simulink model "Drone_Model"  (R2019b)
settings: Solver=VariableStepAuto  StartTime=0.0  StopTime=1  RelTol=1e-3
values from neighbouring files (symbols this model uses):
  A = double(round(subs(J_x,   [states, inputs], [trim_state, trim_input])*1000)/1000)    [state_decoupling.m]
  A_double = [0 1; 0 0]    [kalman_matrices_calculator.m]
  A_s_double = eval(subs(Ad_double,Ts))    [kalman_matrices_calculator.m]
  A_s_single = eval(subs(Ad_single,Ts))    [kalman_matrices_calculator.m]
  A_single = [0]    [kalman_matrices_calculator.m]
  Aaileron = A(5:8,5:8)    [state_decoupling.m]
  Aelevator = A(1:4,1:4)    [state_decoupling.m]
  Arudder = A(11:12,11:12)    [state_decoupling.m]
  Athrust = A(9:10,9:10)    [state_decoupling.m]
  B = B*MotorMix    [state_decoupling.m]
  B_double = [0; 1]    [kalman_matrices_calculator.m]
  B_s_double = eval(subs(Bd_double,Ts))    [kalman_matrices_calculator.m]
  B_s_single = eval(subs(Bd_single,Ts))    [kalman_matrices_calculator.m]
  B_single = [1]    [kalman_matrices_calculator.m]
  Baileron = B(5:8,3)    [state_decoupling.m]
  Belevator = B(1:4,2)    [state_decoupling.m]
  Brudder = B(11:12,4)    [state_decoupling.m]
  Bthrust = B(9:10,1)    [state_decoupling.m]
  C = double(round(subs(J_y,   [states, inputs], [trim_state, trim_input])*1000)/1000)    [state_decoupling.m]
  C_double = [1 0]    [kalman_matrices_calculator.m]
  C_P = 0.041    [state_decoupling.m]
  C_rollpitch = rho*prop_dia^4*prop_dist/sqrt(2)*[                 1  -1  -1   1 ;                 1   1  -1  -1 ;                 0   0   0   0 ; ]    [state_decoupling.m]
  C_single = [1]    [kalman_matrices_calculator.m]
  C_T = [0.069075;4.95e-05]    [state_decoupling.m]
  C_yaw = rho*prop_dia^5/(2*pi)*[                 0   0   0   0 ;                 0   0   0   0 ;                -1   1  -1   1 ; ]    [state_decoupling.m]
  Caileron = [0 1 0 0; 0 0 0 1]    [state_decoupling.m]
  Celevator = [0 1 0 0; 0 0 0 1]    [state_decoupling.m]
  Crudder = [0 1]    [state_decoupling.m]
  Cthrust = [ 1 0; 0 0]    [state_decoupling.m]
  D = D*MotorMix    [state_decoupling.m]
  D_double = [0]    [kalman_matrices_calculator.m]
  D_single = [0]    [kalman_matrices_calculator.m]
  Daileron = [0 ; 0]    [state_decoupling.m]
  Delevator = [0 ; 0]    [state_decoupling.m]
  Drudder = 0    [state_decoupling.m]
  Dthrust = [0 ; D(4,1)]    [state_decoupling.m]
  g = [0;0;UAV_mass*9.81]    [state_decoupling.m]
  J = [      Jxx   0   0 ;       0   Jyy  0 ;       0    0  Jzz; ]    [state_decoupling.m]
  Jinv = inv(J)    [state_decoupling.m]
  L_double = lqe(A_double, G_double, C_double, q_double, r_double, 0)    [kalman_matrices_calculator.m]
  L_single = lqe(A_single, G_single, C_single, q_single, r_single, 0)    [kalman_matrices_calculator.m]
  measurement_noise = 0.1    [kalman_matrices_calculator.m]
  MotorMix = [                 1  1  1 -1 ;                 1  1 -1  1 ;                 1 -1 -1 -1 ;                 1 -1  1  1 ; ]    [state_decoupling.m]
  omega_c = 2*pi*20    (= 125.663706144)    [kalman_matrices_calculator.m]
  process_noise = 0.05    [kalman_matrices_calculator.m]
  Prop_H = 2*pi*Jprop*[               0  0  0  0 ;               0  0  0  0 ;               1 -1  1 -1 ; ]    [state_decoupling.m]
  q_single = cov(out.In_Out_Data{1}.Values.Data)*10000000000000    [kalman_matrices_calculator.m]
  r_single = cov(out.In_Out_Data{2}.Values.Data)    [kalman_matrices_calculator.m]
  Thrust_Sum = rho*prop_dia^4*[                 0   0   0   0 ;                 0   0   0   0 ;                -1  -1  -1  -1 ; ]    [state_decoupling.m]
  trim_input = [293,293,293,293]    [state_decoupling.m]
  trim_state = [0,0,0,0,0,0,0,0,0,0,0,0]    [state_decoupling.m]
  Ts = 0.005    [kalman_matrices_calculator.m]
  UAV_mass = 0.068    [state_decoupling.m]
undefined symbols (not defined in the file or in its folder): DiscIntNeverNeededParam, Discrete, Time
libraries: ctrlSharedLib x10, simulink x3, vrlib x3, dspmtrx3 x1
settings Model: Creator=crbon  LastModifiedBy=Chris

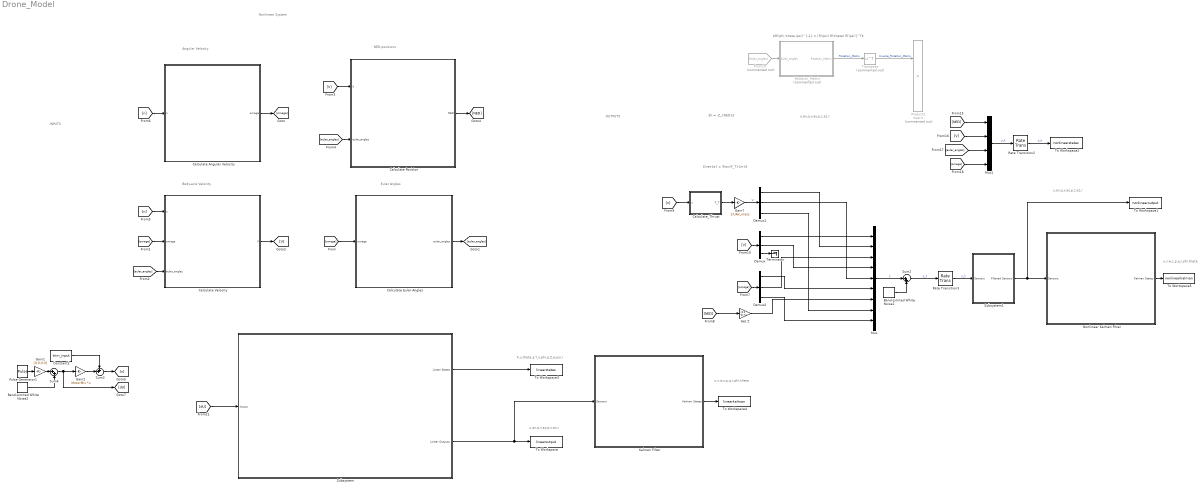
== system Drone_Model ==
  note: X,u,theta,q,Y,v,phi,p,Z,w,psi,r
  note: Nonlinear System
  note: Euler Angles
  note: NED positions
  note: $\vec{a} = \frac{F_T}{m}$
  note: $h = -Z_{NED}$
  note: OUTPUTS
  note: INPUTS
  note: Angular Velocity
  note: Body-axis Velocity
  note: u,ax,q,v,ay,p,z,az,r
  note: u,v,w,z,p,q,r,phi,theta
  note: u,ax,q,v,ay,p,z,az,r
  note: $R(\phi,\theta,\psi)^{-1} = [R(\psi) R(\theta) R(\psi)]^T$
  note: u,v,w,z,p,q,r,phi,theta
  note: u,ax,q,v,ay,p,z,az,r
  Band-Limited White Noise1 : simulink/Sources/Band-Limited White Noise  Cov=measurement_noise*ones(9,1)  Ts=0.05  seed=[11;12;13;14;15;16;17;18;19]
  Band-Limited White Noise2 : simulink/Sources/Band-Limited White Noise  Cov=process_noise*ones(4,1)  Ts=0.05  seed=[1;2;3;4]
  Calculate Angular Velocity : Subsystem
  Calculate Euler Angles : Subsystem
  Calculate Position : Subsystem
  Calculate Velocity : Subsystem
  Calculate_Thrust : Subsystem
  Constant2 : Constant  Value=trim_input
  Demux : Demux  Outputs=3
  Demux1 : Demux  Outputs=3
  Demux2 : Demux  Outputs=3
  From19 : From  Commented=on  GotoTag=euler_angles
  Gain1 : Gain  Gain=[0;0;0;0]
      settings: AttributesFormatString=%<Gain>
  Gain2 : Gain  Gain=MotorMix  Multiplication=Matrix(K*u)
      settings: AttributesFormatString=%<Gain>
  Gain7 : Gain  Gain=1/UAV_mass
      settings: AttributesFormatString=%<Gain>
  Get Z : Gain  Gain=[0 0 -1]  Multiplication=Matrix(K*u)
  Kalman Filter : Subsystem
  Mux : Mux  Inputs=9
  Mux1 : Mux
  Nonlinear Kalman Filter : Subsystem
  Product2 : Product  Commented=on  Multiplication=Matrix(*)
  Pulse Generator1 : DiscretePulseGenerator  PulseType=Time based  Amplitude=0.05  Period=10  PulseWidth=40  PhaseDelay=1
  Rate Transition2 : RateTransition  OutPortSampleTime=0.005
  Rate Transition3 : RateTransition  OutPortSampleTime=0.005
  Rotation_Matrix : Subsystem  Commented=on
  Subsystem : Subsystem
  Subsystem1 : Subsystem
  Sum2 : Sum  Inputs=|++
  Sum3 : Sum  Inputs=++|
  Sum4 : Sum  Inputs=|++
  Terminator : Terminator
  To Workspace : ToWorkspace  VariableName=linearoutput  SaveFormat=Timeseries  SampleTime=-1
  To Workspace1 : ToWorkspace  VariableName=nonlinearoutput  SaveFormat=Timeseries  SampleTime=-1
  To Workspace2 : ToWorkspace  VariableName=nonlinearstates  SaveFormat=Timeseries  SampleTime=-1
  To Workspace3 : ToWorkspace  VariableName=linearstates  SaveFormat=Timeseries  SampleTime=-1
  To Workspace4 : ToWorkspace  VariableName=linearkalman  SaveFormat=Timeseries  SampleTime=-1
  To Workspace5 : ToWorkspace  VariableName=nonlinearkalman  SaveFormat=Timeseries  SampleTime=-1
  Transpose : Math  Commented=on  Operator=transpose  SignedPower=off  SaturateOnIntegerOverflow=on
  wires:
  [omega] -> Calculate Euler Angles/1(omega)
  Calculate Angular Velocity/1(omega) -> [omega]
  [omega] -> Calculate Velocity/2(omega)
  Calculate Euler Angles/1(euler_angles) -> [euler_angles]
  [euler_angles] -> Calculate Velocity/3(euler_angles)
  Calculate Velocity/1(V) -> [V]
  [V] -> Calculate Position/1("V ")
  [euler_angles] -> Calculate Position/2(euler_angles)
  [n] -> Calculate Velocity/1(n)
  [n] -> Calculate Angular Velocity/1(n)
  Calculate Position/1(NED) -> [NED]
  [NED] -> Get Z/1
  Get Z/1 -> Mux/7
  [dU] -> Subsystem/1("Inputs ")
  Subsystem/1(Linear States) -> To Workspace3/1
  Subsystem/2(Linear Outputs) -> Kalman Filter/1(Sensors), To Workspace/1
  Kalman Filter/1(Kalman States) -> To Workspace4/1
  Rotation_Matrix/1(Rotation_Matrix) -> Transpose/1  "Rotation_Matrix"
  From19/1 -> Rotation_Matrix/1("euler_angles ")
  Transpose/1 -> Product2/1  "Inverse_Rotation_Matrix"
  Calculate_Thrust/1(F_T) -> Gain7/1
  [n] -> Calculate_Thrust/1(n)
  Gain7/1 -> Demux1/1  "V"
  [NED] -> Mux1/1
  [euler_angles] -> Mux1/3
  [omega] -> Mux1/4
  [V] -> Mux1/2
  [V] -> Demux/1
  Demux/3 -> Terminator/1
  Demux/1 -> Mux/1
  Demux/2 -> Mux/4
  Demux1/1 -> Mux/2
  Demux1/2 -> Mux/5
  Demux1/3 -> Mux/8
  [omega] -> Demux2/1
  Demux2/1 -> Mux/6
  Demux2/2 -> Mux/3
  Demux2/3 -> Mux/9
  Nonlinear Kalman Filter/1(Kalman States) -> To Workspace5/1
  Mux1/1 -> Rate Transition2/1  "y_k"
  Sum2/1 -> Rate Transition3/1  "y_k"
  Mux/1 -> Sum2/1  "y"
  Rate Transition2/1 -> To Workspace2/1  "y_k"
  Rate Transition3/1 -> Subsystem1/1(Sensors)  "y_k"
  Band-Limited White Noise1/1 -> Sum2/2
  Subsystem1/1(Filtered Sensors) -> Nonlinear Kalman Filter/1(Sensors), To Workspace1/1
  Gain1/1 -> Sum4/1
  Band-Limited White Noise2/1 -> Sum4/2
  Pulse Generator1/1 -> Gain1/1
  Gain2/1 -> Sum3/2
  Sum3/1 -> [n]
  Sum4/1 -> Gain2/1, [dU]
  Constant2/1 -> Sum3/1

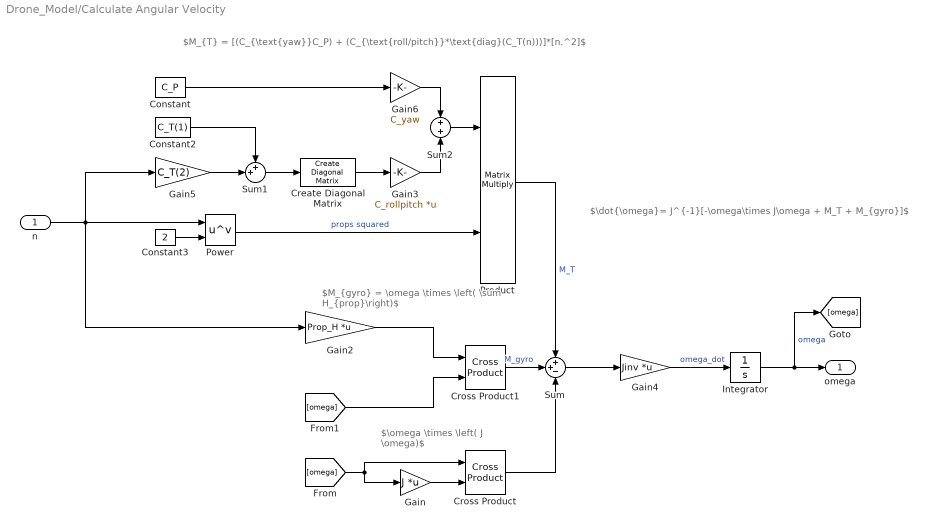
== system Drone_Model/Calculate Angular Velocity ==
  note: $M_{gyro} = \omega \times \left( \sum H_{prop}\right)$
  note: $\dot{\omega}= J^{-1}[-\omega\times J\omega + M_T + M_{gyro}]$
  note: $\omega \times \left( J \omega)$
  note: $M_{T} = [(C_{\text{yaw}}C_P) + (C_{\text{roll/pitch}}*\text{diag}(C_T(n)))]*[n.^2]$
  n : Inport
  Constant : Constant  Value=C_P
  Constant2 : Constant  Value=C_T(1)
  Constant3 : Constant  Value=2
  Create Diagonal Matrix : dspmtrx3/Create Diagonal Matrix
      settings: SourceProductName=DSP System Toolbox  SourceProductBaseCode=DS
  Cross Product : vrlib/Utilities/Cross Product
      settings: SourceProductName=Simulink
  Cross Product1 : vrlib/Utilities/Cross Product
      settings: SourceProductName=Simulink
  Gain : Gain  Gain=J  Multiplication=Matrix(K*u)
  Gain2 : Gain  Gain=Prop_H  Multiplication=Matrix(K*u)
  Gain3 : Gain  Gain=C_rollpitch  Multiplication=Matrix(K*u)
      settings: AttributesFormatString=%<Gain>
  Gain4 : Gain  Gain=Jinv  Multiplication=Matrix(K*u)
      settings: AttributesFormatString=%<Gain>
  Gain5 : Gain  Gain=C_T(2)
  Gain6 : Gain  Gain=C_yaw
      settings: AttributesFormatString=%<Gain>
  Integrator : Integrator  InitialCondition=[0;0;0]
  Power : Math  Operator=pow  SignedPower=off  SaturateOnIntegerOverflow=on
  Product : Product  Multiplication=Matrix(*)
  Sum : Sum  Inputs=++-
  Sum1 : Sum  Inputs=++|
  Sum2 : Sum  Inputs=+|+
  omega : Outport
  wires:
  Sum/1 -> Gain4/1
  [omega] -> Gain/1, Cross Product/1
  Cross Product/1 -> Sum/3
  [omega] -> Cross Product1/2
  Gain2/1 -> Cross Product1/1
  Cross Product1/1 -> Sum/2  "M_gyro"
  Gain4/1 -> Integrator/1  "omega_dot"
  Gain/1 -> Cross Product/2
  Integrator/1 -> [omega], omega/1  "omega"
  Product/1 -> Sum/1  "M_T"
  Create Diagonal Matrix/1 -> Gain3/1
  Sum2/1 -> Product/1
  Sum1/1 -> Create Diagonal Matrix/1
  Constant/1 -> Gain6/1
  Power/1 -> Product/2  "props squared"
  Gain6/1 -> Sum2/1
  Gain5/1 -> Sum1/2
  Gain3/1 -> Sum2/2
  n/1 -> Gain2/1, Power/1, Gain5/1
  Constant2/1 -> Sum1/1
  Constant3/1 -> Power/2

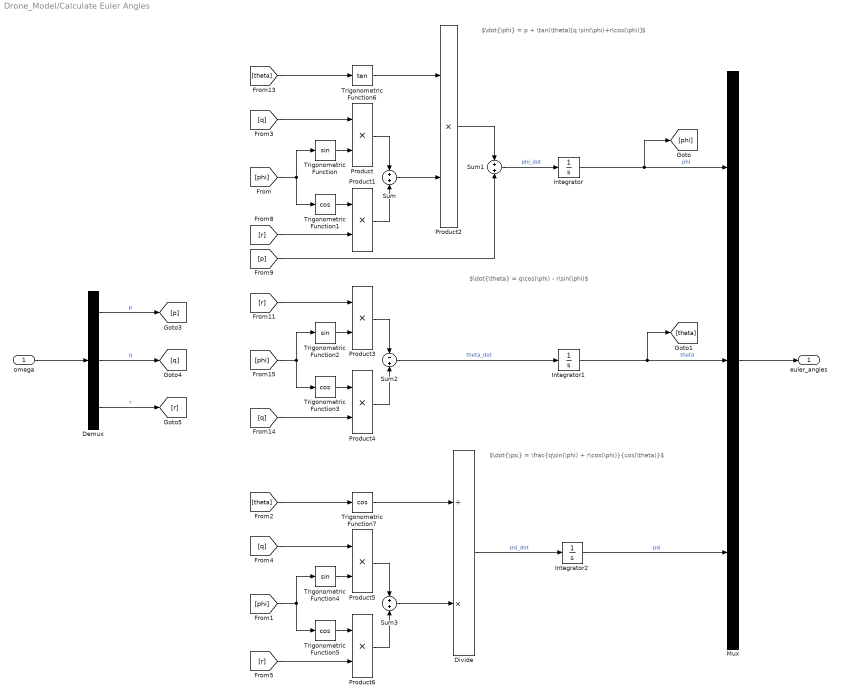
== system Drone_Model/Calculate Euler Angles ==
  note: $\dot{\phi} = p + \tan(\theta)[q \sin(\phi)+r\cos(\phi)]$
  note: $\dot{\theta} = q\cos(\phi) - r\sin(\phi)$
  note: $\dot{\psi} = \frac{q\sin(\phi) + r\cos(\phi)}{cos(\theta)}$
  omega : Inport
  Demux : Demux  Outputs=3
  Divide : Product  Inputs=/*
  Integrator : Integrator
  Integrator1 : Integrator
  Integrator2 : Integrator
  Mux : Mux  Inputs=3
  Product{,1..6} (7 alike) : Product
  Sum : Sum  Inputs=+|+
  Sum1 : Sum  Inputs=+|+
  Sum2 : Sum  Inputs=-|+
  Sum3 : Sum  Inputs=+|+
  Trigonometric Function : Trigonometry
  Trigonometric Function{1,3,5,7} (4 alike) : Trigonometry  Operator=cos
  Trigonometric Function2 : Trigonometry
  Trigonometric Function4 : Trigonometry
  Trigonometric Function6 : Trigonometry  Operator=tan
  euler_angles : Outport
  wires:
  Trigonometric Function7/1 -> Divide/1
  Product1/1 -> Sum/2
  Product6/1 -> Sum3/2
  Trigonometric Function/1 -> Product/2
  Product5/1 -> Sum3/1
  [theta] -> Trigonometric Function7/1
  Trigonometric Function6/1 -> Product2/1
  [r] -> Product6/2
  [theta] -> Trigonometric Function6/1
  Integrator1/1 -> [theta], Mux/2  "theta"
  Trigonometric Function4/1 -> Product5/2
  [q] -> Product4/2
  Demux/3 -> [r]  "r"
  Divide/1 -> Integrator2/1  "psi_dot"
  Integrator2/1 -> Mux/3  "psi"
  [q] -> Product5/1
  Product4/1 -> Sum2/2
  [q] -> Product/1
  [phi] -> Trigonometric Function4/1, Trigonometric Function5/1
  Sum2/1 -> Integrator1/1  "theta_dot"
  Trigonometric Function5/1 -> Product6/1
  Trigonometric Function3/1 -> Product4/1
  [r] -> Product3/1
  Integrator/1 -> [phi], Mux/1  "phi"
  Sum3/1 -> Divide/2
  Product3/1 -> Sum2/1
  [phi] -> Trigonometric Function2/1, Trigonometric Function3/1
  Demux/1 -> [p]  "p"
  Product2/1 -> Sum1/1
  [r] -> Product1/2
  Trigonometric Function1/1 -> Product1/1
  [phi] -> Trigonometric Function1/1, Trigonometric Function/1
  omega/1 -> Demux/1
  Product/1 -> Sum/1
  Demux/2 -> [q]  "q"
  Sum/1 -> Product2/2
  Mux/1 -> euler_angles/1
  Sum1/1 -> Integrator/1  "phi_dot"
  [p] -> Sum1/2
  Trigonometric Function2/1 -> Product3/2

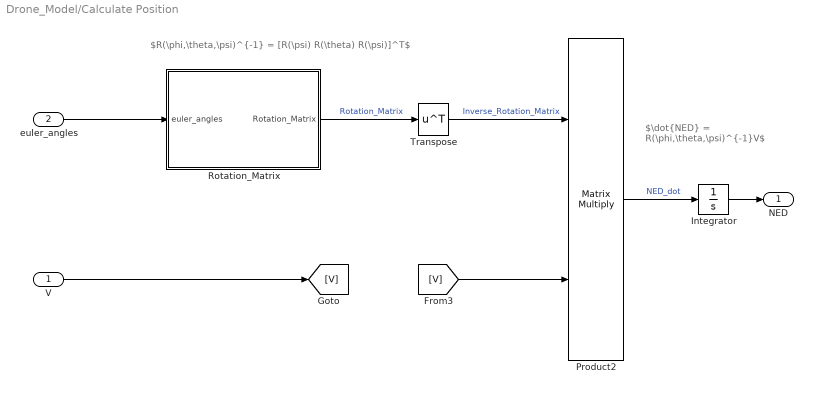
== system Drone_Model/Calculate Position ==
  note: $R(\phi,\theta,\psi)^{-1} = [R(\psi) R(\theta) R(\psi)]^T$
  note: $\dot{NED} = R(\phi,\theta,\psi)^{-1}V$
  "V " : Inport
  euler_angles : Inport  Port=2
  Integrator : Integrator  InitialCondition=[0;0;0]
  Product2 : Product  Multiplication=Matrix(*)
  Rotation_Matrix : Subsystem
  Transpose : Math  Operator=transpose  SignedPower=off  SaturateOnIntegerOverflow=on
  NED : Outport
  wires:
  Product2/1 -> Integrator/1  "NED_dot"
  "V "/1 -> [V]
  Rotation_Matrix/1(Rotation_Matrix) -> Transpose/1  "Rotation_Matrix"
  Transpose/1 -> Product2/1  "Inverse_Rotation_Matrix"
  [V] -> Product2/2
  euler_angles/1 -> Rotation_Matrix/1("euler_angles ")
  Integrator/1 -> NED/1

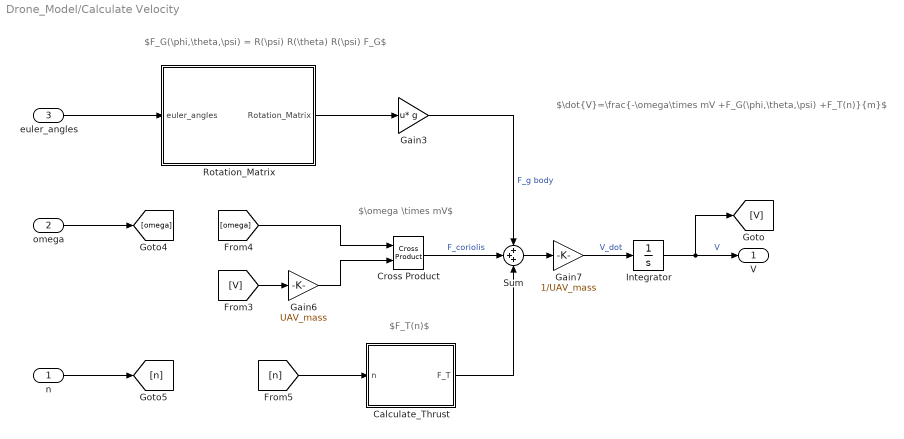
== system Drone_Model/Calculate Velocity ==
  note: $F_G(\phi,\theta,\psi) = R(\psi) R(\theta) R(\psi) F_G$
  note: $\dot{V}=\frac{-\omega\times mV +F_G(\phi,\theta,\psi) +F_T(n)}{m}$
  note: $\omega \times mV$
  note: $F_T(n)$
  n : Inport
  omega : Inport  Port=2
  euler_angles : Inport  Port=3
  Calculate_Thrust : Subsystem
  Cross Product : vrlib/Utilities/Cross Product
      settings: SourceProductName=Simulink
  Gain3 : Gain  Gain=g  Multiplication=Matrix(u*K)
      settings: AttributesFormatString=%<Gain>
  Gain6 : Gain  Gain=UAV_mass
      settings: AttributesFormatString=%<Gain>
  Gain7 : Gain  Gain=1/UAV_mass
      settings: AttributesFormatString=%<Gain>
  Integrator : Integrator  InitialCondition=[0;0;0]
  Rotation_Matrix : Subsystem
  Sum : Sum  Inputs=+++
  V : Outport
  wires:
  [V] -> Gain6/1
  [omega] -> Cross Product/1
  Cross Product/1 -> Sum/2  "F_coriolis"
  Gain3/1 -> Sum/1  "F_g body"
  Gain6/1 -> Cross Product/2
  Sum/1 -> Gain7/1
  Integrator/1 -> V/1, [V]  "V"
  omega/1 -> [omega]
  n/1 -> [n]
  Rotation_Matrix/1(Rotation_Matrix) -> Gain3/1
  euler_angles/1 -> Rotation_Matrix/1("euler_angles ")
  [n] -> Calculate_Thrust/1(n)
  Gain7/1 -> Integrator/1  "V_dot"
  Calculate_Thrust/1(F_T) -> Sum/3

== system Drone_Model/Calculate_Thrust ==
  note: $F_{T} = \sum_{i=1}^4[0;0;C_{T}.*n.^2]$
  n : Inport
  Constant15 : Constant  Value=C_T(1)
  Constant16 : Constant  Value=2
  Gain4 : Gain  Gain=Thrust_Sum  Multiplication=Matrix(K*u)
      settings: AttributesFormatString=%<Gain>
  Gain5 : Gain  Gain=C_T(2)
  Power : Math  Operator=pow  SignedPower=off  SaturateOnIntegerOverflow=on
  Product2 : Product
  Sum1 : Sum  Inputs=++|
  F_T : Outport
  wires:
  Constant15/1 -> Sum1/1
  Gain4/1 -> F_T/1  "F_T"
  n/1 -> Power/1, Gain5/1
  Power/1 -> Product2/2  "props squared"
  Gain5/1 -> Sum1/2
  Sum1/1 -> Product2/1
  Product2/1 -> Gain4/1
  Constant16/1 -> Power/2

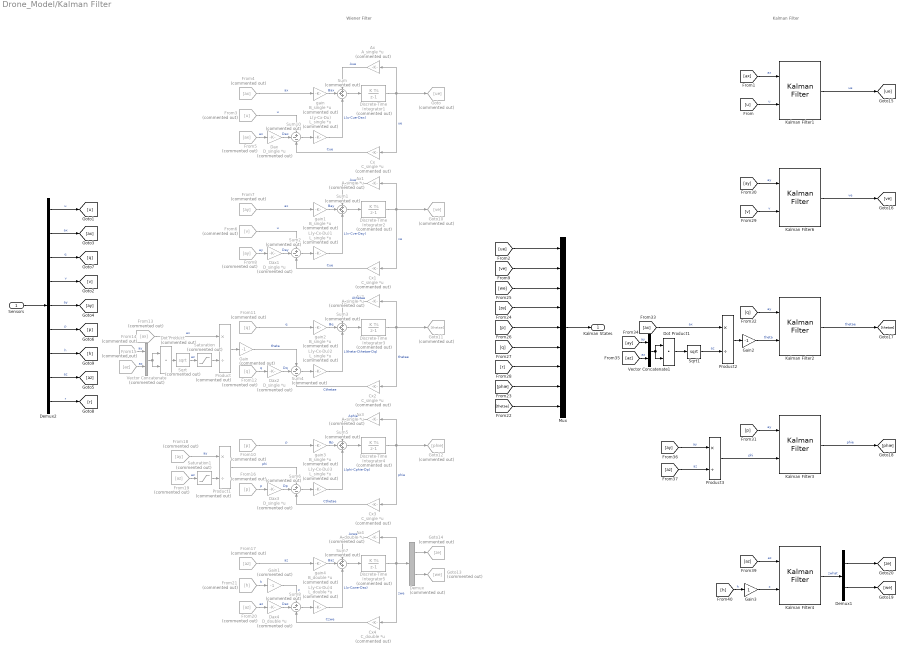
== system Drone_Model/Kalman Filter ==
  note: Wiener Filter
  note: Kalman Filter
  Sensors : Inport
  Ax{,1..3} (4 alike) : Gain  Commented=on  Gain=A_single  Multiplication=Matrix(K*u)
      settings: AttributesFormatString=Ax
  Ax4 : Gain  Commented=on  Gain=A_double  Multiplication=Matrix(K*u)
      settings: AttributesFormatString=Ax
  Cx{,1..3} (4 alike) : Gain  Commented=on  Gain=C_single  Multiplication=Matrix(K*u)
      settings: AttributesFormatString=Cx
  Cx4 : Gain  Commented=on  Gain=C_double  Multiplication=Matrix(K*u)
      settings: AttributesFormatString=Cx
  Dax{,1..3} (4 alike) : Gain  Commented=on  Gain=D_single  Multiplication=Matrix(K*u)
      settings: AttributesFormatString=Du
  Dax4 : Gain  Commented=on  Gain=D_double  Multiplication=Matrix(K*u)
      settings: AttributesFormatString=Du
  Demux : Demux  Commented=on  Outputs=2
  Demux1 : Demux  Outputs=2
  Demux2 : Demux  Outputs=9
  Discrete-Time Integrator{1..5} (5 alike) : DiscreteIntegrator  Commented=on  SampleTime=-1  ICPrevOutput=DiscIntNeverNeededParam  ICPrevScaledInput=DiscIntNeverNeededParam
  Dot Product : DotProduct  Commented=on  OutMin=0.0001  InputSameDT=on  OutDataTypeStr=Inherit: Inherit via internal rule
  Dot Product1 : DotProduct  OutMin=0.0001  InputSameDT=on  OutDataTypeStr=Inherit: Inherit via internal rule
  From10 : From  Commented=on  GotoTag=p
  From11 : From  Commented=on  GotoTag=q
  From12 : From  Commented=on  GotoTag=q
  From13 : From  Commented=on  GotoTag=ax
  From{7..8,14,18} (4 alike) : From  Commented=on  GotoTag=ay
  From{15,17,19..20} (4 alike) : From  Commented=on  GotoTag=az
  From16 : From  Commented=on  GotoTag=p
  From21 : From  Commented=on  GotoTag=h
  From3 : From  Commented=on  GotoTag=u
  From4 : From  Commented=on  GotoTag=ax
  From5 : From  Commented=on  GotoTag=ax
  From6 : From  Commented=on  GotoTag=v
  Gain : Gain  Commented=on  Gain=-1
  Gain1 : Gain  Commented=on  Gain=-1
  Gain2 : Gain  Gain=-1
  Gain3 : Gain
  Goto : Goto  Commented=on  GotoTag=ue
  Goto10 : Goto  Commented=on  GotoTag=ve
  Goto11 : Goto  Commented=on  GotoTag=thetae
  Goto12 : Goto  Commented=on  GotoTag=phie
  Goto13 : Goto  Commented=on  GotoTag=we
  Goto14 : Goto  Commented=on  GotoTag=ze
  Kalman Filter{1..3,6} (4 alike) : ctrlSharedLib/Kalman Filter  TimeDomain=Discrete-Time  UseCurrentEstimator=on  ModelSource=Individual A, B, C, D matrices  ModelSourceVariable=ss(0.95,1,1,0,1)  A=A_s_single  B=B_s_single  C=C_single  D=D_single  NumberOfStates=1  NumberOfInputs=1  NumberOfOutputs=1  InitialEstimateSource=Dialog  X0=[0]  P0=10  UseK=off  UseGH=off  NumberOfProcessNoiseInputs=1  G=1  TimeInvariantG=on  H=0  TimeInvariantH=on  Q=[1]*q_single  TimeInvariantQ=on  R=[1]*r_single  TimeInvariantR=on  N=0  TimeInvariantN=on  AddInputPort=on  AddEnablePort=off  OutputEstimatedY=off  OutputP=off  Ts=Ts
      settings: SourceProductBaseCode=CT
  Kalman Filter4 : ctrlSharedLib/Kalman Filter  TimeDomain=Discrete-Time  UseCurrentEstimator=on  ModelSource=Individual A, B, C, D matrices  ModelSourceVariable=ss(0.95,1,1,0,1)  A=A_s_double  B=B_s_double  C=C_double  D=D_double  NumberOfStates=1  NumberOfInputs=1  NumberOfOutputs=1  InitialEstimateSource=Dialog  X0=[0]  P0=10  UseK=off  UseGH=off  NumberOfProcessNoiseInputs=1  G=1  TimeInvariantG=on  H=0  TimeInvariantH=on  Q=[0 0 ; 0 1]*q_single  TimeInvariantQ=on  R=[1]*r_single  TimeInvariantR=on  N=0  TimeInvariantN=on  AddInputPort=on  AddEnablePort=off  OutputEstimatedY=off  OutputP=off  Ts=Ts
      settings: SourceProductBaseCode=CT
  L(y-Cx-Du){,1..3} (4 alike) : Gain  Commented=on  Gain=L_single  Multiplication=Matrix(K*u)
      settings: AttributesFormatString=L(y-Cx-Du)
  L(y-Cx-Du)4 : Gain  Commented=on  Gain=L_double  Multiplication=Matrix(K*u)
      settings: AttributesFormatString=L(y-Cx-Du)
  Mux : Mux  Inputs=9
  Product : Product  Commented=on  Inputs=*/
  Product1 : Product  Commented=on  Inputs=*/
  Product2 : Product  Inputs=*/
  Product3 : Product  Inputs=*/
  Saturation : Saturate  Commented=on  UpperLimit=inf  LowerLimit=0.001
  Saturation1 : Saturate  Commented=on  UpperLimit=inf  LowerLimit=0.001
  Sqrt : Sqrt  Commented=on  SaturateOnIntegerOverflow=on
  Sqrt1 : Sqrt  SaturateOnIntegerOverflow=on
  Sum{,1,3,5,7} (5 alike) : Sum  Commented=on  Inputs=+++
  Sum{2,4,6,8,10} (5 alike) : Sum  Commented=on  Inputs=+--
  Vector Concatenate : Concatenate  Commented=on
  Vector Concatenate1 : Concatenate
  gain{,1..3} (4 alike) : Gain  Commented=on  Gain=B_single  Multiplication=Matrix(K*u)
      settings: AttributesFormatString=Bu
  gain4 : Gain  Commented=on  Gain=B_double  Multiplication=Matrix(K*u)
      settings: AttributesFormatString=Bu
  Kalman States : Outport
  wires:
  Discrete-Time Integrator1/1 -> Goto/1, Cx/1, Ax/1  "ue"
  Sum10/1 -> L(y-Cx-Du)/1
  Ax/1 -> Sum/1  "Aue"
  L(y-Cx-Du)/1 -> Sum/3  "L(u-Cue-Dax)"
  Cx/1 -> Sum10/3  "Cue"
  From4/1 -> gain/1  "ax"
  gain/1 -> Sum/2  "Bax"
  From3/1 -> Sum10/1  "u"
  From5/1 -> Dax/1  "ax"
  Dax/1 -> Sum10/2  "Dax"
  Sum/1 -> Discrete-Time Integrator1/1
  Demux2/1 -> [u]  "u"
  Sensors/1 -> Demux2/1
  Demux2/6 -> [p]  "p"
  Sum1/1 -> Discrete-Time Integrator2/1
  Dax1/1 -> Sum2/2  "Day"
  From8/1 -> Dax1/1  "ay"
  From6/1 -> Sum2/1  "u"
  gain1/1 -> Sum1/2  "Bay"
  From7/1 -> gain1/1  "ax"
  Cx1/1 -> Sum2/3  "Cue"
  L(y-Cx-Du)1/1 -> Sum1/3  "L(v-Cve-Day)"
  Ax1/1 -> Sum1/1  "Aue"
  Sum2/1 -> L(y-Cx-Du)1/1
  Discrete-Time Integrator2/1 -> Ax1/1, Cx1/1, Goto10/1  "ve"
  Discrete-Time Integrator3/1 -> Goto11/1, Cx2/1, Ax2/1  "thetae"
  Sum4/1 -> L(y-Cx-Du)2/1
  Ax2/1 -> Sum3/1  "Athetae"
  L(y-Cx-Du)2/1 -> Sum3/3  "L(theta-Cthetae-Dq)"
  Cx2/1 -> Sum4/3  "Cthetae"
  From11/1 -> gain2/1  "q"
  gain2/1 -> Sum3/2  "Bq"
  Gain/1 -> Sum4/1  "theta"
  From12/1 -> Dax2/1  "q"
  Dax2/1 -> Sum4/2  "Dq"
  Sum3/1 -> Discrete-Time Integrator3/1
  From14/1 -> Vector Concatenate/1  "ay"
  From15/1 -> Vector Concatenate/2  "az"
  Vector Concatenate/1 -> Dot Product/1, Dot Product/2
  Dot Product/1 -> Sqrt/1
  From13/1 -> Product/1  "ax"
  Product/1 -> Gain/1
  From18/1 -> Product1/1  "ay"
  Sum5/1 -> Discrete-Time Integrator4/1
  Dax3/1 -> Sum6/2  "Dp"
  From16/1 -> Dax3/1  "p"
  Product1/1 -> Sum6/1  "phi"
  gain3/1 -> Sum5/2  "Bp"
  From10/1 -> gain3/1  "p"
  Cx3/1 -> Sum6/3  "Cthetae"
  L(y-Cx-Du)3/1 -> Sum5/3  "L(phi-Cphie-Dp)"
  Ax3/1 -> Sum5/1  "Aphie"
  Sum6/1 -> L(y-Cx-Du)3/1
  Discrete-Time Integrator4/1 -> Ax3/1, Cx3/1, Goto12/1  "phie"
  Discrete-Time Integrator5/1 -> Ax4/1, Demux/1, Cx4/1  "zwe"
  Sum8/1 -> L(y-Cx-Du)4/1
  Ax4/1 -> Sum7/1  "Azwe"
  L(y-Cx-Du)4/1 -> Sum7/3  "L(z-Czwe-Daz)"
  Cx4/1 -> Sum8/3  "Czwe"
  From17/1 -> gain4/1  "az"
  gain4/1 -> Sum7/2  "Baz"
  From21/1 -> Gain1/1  "h"
  From20/1 -> Dax4/1  "az"
  Dax4/1 -> Sum8/2  "Daz"
  Sum7/1 -> Discrete-Time Integrator5/1
  Demux/2 -> Goto13/1
  Demux/1 -> Goto14/1
  Gain1/1 -> Sum8/1  "z"
  [ue] -> Mux/1
  [ve] -> Mux/2
  [we] -> Mux/3
  [ze] -> Mux/4
  Mux/1 -> Kalman States/1
  [r] -> Mux/7
  [q] -> Mux/6
  [p] -> Mux/5
  [phie] -> Mux/8
  [thetae] -> Mux/9
  [ax] -> Kalman Filter1/1  "ax"
  [u] -> Kalman Filter1/2  "u"
  [v] -> Kalman Filter6/2  "v"
  [ay] -> Kalman Filter6/1  "ay"
  [q] -> Kalman Filter2/1  "ay"
  Gain2/1 -> Kalman Filter2/2  "theta"
  Sqrt/1 -> Saturation/1  "az"
  Saturation/1 -> Product/2
  From19/1 -> Saturation1/1  "az"
  Saturation1/1 -> Product1/2
  Sqrt1/1 -> Product2/2  "az"
  Product2/1 -> Gain2/1
  [ax] -> Product2/1  "ax"
  Dot Product1/1 -> Sqrt1/1
  Vector Concatenate1/1 -> Dot Product1/2, Dot Product1/1
  [az] -> Vector Concatenate1/2  "az"
  [ay] -> Vector Concatenate1/1  "ay"
  [p] -> Kalman Filter3/1  "ay"
  [az] -> Product3/2  "az"
  Product3/1 -> Kalman Filter3/2  "phi"
  [ay] -> Product3/1  "ay"
  Kalman Filter4/1 -> Demux1/1  "zwhat"
  [az] -> Kalman Filter4/1  "az"
  Gain3/1 -> Kalman Filter4/2  "z"
  Demux1/1 -> [ze]
  Demux1/2 -> [we]
  Kalman Filter3/1 -> [phie]  "phie"
  Kalman Filter2/1 -> [thetae]  "thetae"
  Kalman Filter6/1 -> [ve]  "ve"
  Kalman Filter1/1 -> [ue]  "ue"
  [h] -> Gain3/1  "h"
  Demux2/2 -> [ax]  "ax"
  Demux2/4 -> [v]  "v"
  Demux2/3 -> [q]  "q"
  Demux2/8 -> [az]  "az"
  Demux2/5 -> [ay]  "ay"
  Demux2/7 -> [h]  "h"
  Demux2/9 -> [r]  "r"

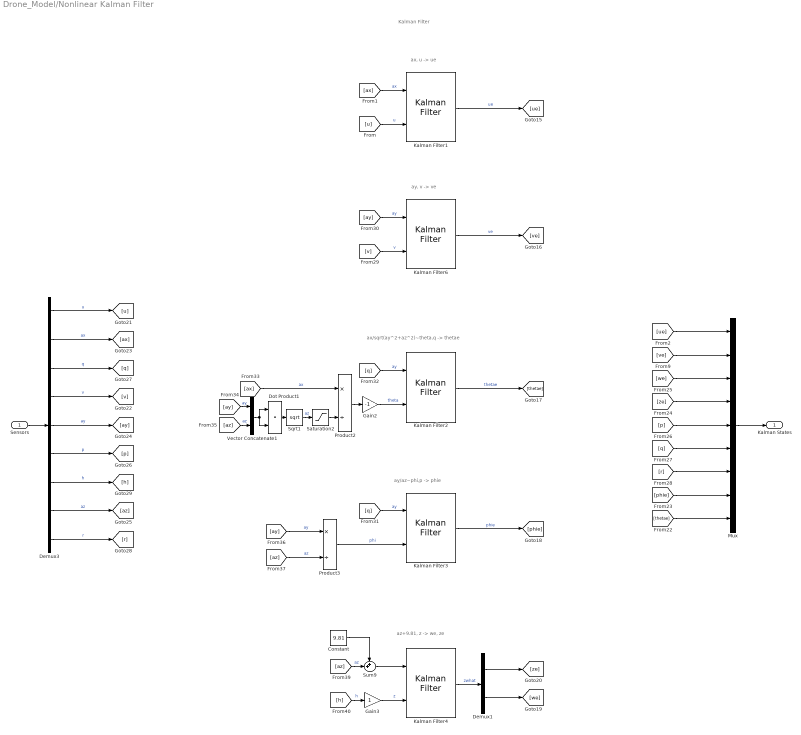
== system Drone_Model/Nonlinear Kalman Filter ==
  note: Kalman Filter
  note: ay, v -> ve
  note: ax, u -> ue
  note: ax/sqrt(ay^2+az^2)~theta,q -> thetae
  note: ay/az~phi,p -> phie
  note: az+9.81, z -> we, ze
  Sensors : Inport
  Constant : Constant  Value=9.81
  Demux1 : Demux  Outputs=2
  Demux3 : Demux  Outputs=9
  Dot Product1 : DotProduct  OutMin=0.0001  InputSameDT=on  OutDataTypeStr=Inherit: Inherit via internal rule
  Gain2 : Gain  Gain=-1
  Gain3 : Gain
  Kalman Filter{1..3,6} (4 alike) : ctrlSharedLib/Kalman Filter  TimeDomain=Discrete-Time  UseCurrentEstimator=on  ModelSource=Individual A, B, C, D matrices  ModelSourceVariable=ss(0.95,1,1,0,1)  A=A_s_single  B=B_s_single  C=C_single  D=D_single  NumberOfStates=1  NumberOfInputs=1  NumberOfOutputs=1  InitialEstimateSource=Dialog  X0=[0]  P0=10  UseK=off  UseGH=off  NumberOfProcessNoiseInputs=1  G=1  TimeInvariantG=on  H=0  TimeInvariantH=on  Q=[1]*q_single  TimeInvariantQ=on  R=[1]*r_single*10000  TimeInvariantR=on  N=0  TimeInvariantN=on  AddInputPort=on  AddEnablePort=off  OutputEstimatedY=off  OutputP=off  Ts=Ts
      settings: SourceProductBaseCode=CT
  Kalman Filter4 : ctrlSharedLib/Kalman Filter  TimeDomain=Discrete-Time  UseCurrentEstimator=on  ModelSource=Individual A, B, C, D matrices  ModelSourceVariable=ss(0.95,1,1,0,1)  A=A_s_double  B=B_s_double  C=C_double  D=D_double  NumberOfStates=1  NumberOfInputs=1  NumberOfOutputs=1  InitialEstimateSource=Dialog  X0=[0]  P0=10  UseK=off  UseGH=off  NumberOfProcessNoiseInputs=1  G=1  TimeInvariantG=on  H=0  TimeInvariantH=on  Q=[0 0; 0 1]*q_single  TimeInvariantQ=on  R=[1]*r_single*10000  TimeInvariantR=on  N=0  TimeInvariantN=on  AddInputPort=on  AddEnablePort=off  OutputEstimatedY=off  OutputP=off  Ts=Ts
      settings: SourceProductBaseCode=CT
  Mux : Mux  Inputs=9
  Product2 : Product  Inputs=*/
  Product3 : Product  Inputs=*/
  Saturation2 : Saturate  UpperLimit=inf  LowerLimit=0.001
  Sqrt1 : Sqrt  SaturateOnIntegerOverflow=on
  Sum9 : Sum  Inputs=++|
  Vector Concatenate1 : Concatenate
  Kalman States : Outport
  wires:
  [h] -> Gain3/1  "h"
  Kalman Filter1/1 -> [ue]  "ue"
  Kalman Filter6/1 -> [ve]  "ve"
  Kalman Filter2/1 -> [thetae]  "thetae"
  Kalman Filter3/1 -> [phie]  "phie"
  Demux1/2 -> [we]
  Demux1/1 -> [ze]
  Gain3/1 -> Kalman Filter4/2  "z"
  Kalman Filter4/1 -> Demux1/1  "zwhat"
  [ay] -> Product3/1  "ay"
  Product3/1 -> Kalman Filter3/2  "phi"
  [az] -> Product3/2  "az"
  [q] -> Kalman Filter3/1  "ay"
  [ay] -> Vector Concatenate1/1  "ay"
  [az] -> Vector Concatenate1/2  "az"
  Vector Concatenate1/1 -> Dot Product1/1, Dot Product1/2
  Dot Product1/1 -> Sqrt1/1
  [ax] -> Product2/1  "ax"
  Product2/1 -> Gain2/1
  Sqrt1/1 -> Saturation2/1  "az"
  Saturation2/1 -> Product2/2
  Gain2/1 -> Kalman Filter2/2  "theta"
  [q] -> Kalman Filter2/1  "ay"
  [ay] -> Kalman Filter6/1  "ay"
  [v] -> Kalman Filter6/2  "v"
  [u] -> Kalman Filter1/2  "u"
  [ax] -> Kalman Filter1/1  "ax"
  [thetae] -> Mux/9
  [phie] -> Mux/8
  [p] -> Mux/5
  [q] -> Mux/6
  [r] -> Mux/7
  Mux/1 -> Kalman States/1
  [ze] -> Mux/4
  [we] -> Mux/3
  [ve] -> Mux/2
  [ue] -> Mux/1
  [az] -> Sum9/2  "az"
  Sum9/1 -> Kalman Filter4/1
  Constant/1 -> Sum9/1
  Demux3/7 -> [h]  "h"
  Demux3/8 -> [az]  "az"
  Demux3/2 -> [ax]  "ax"
  Demux3/1 -> [u]  "u"
  Demux3/4 -> [v]  "v"
  Sensors/1 -> Demux3/1
  Demux3/3 -> [q]  "q"
  Demux3/6 -> [p]  "p"
  Demux3/5 -> [ay]  "ay"
  Demux3/9 -> [r]  "r"

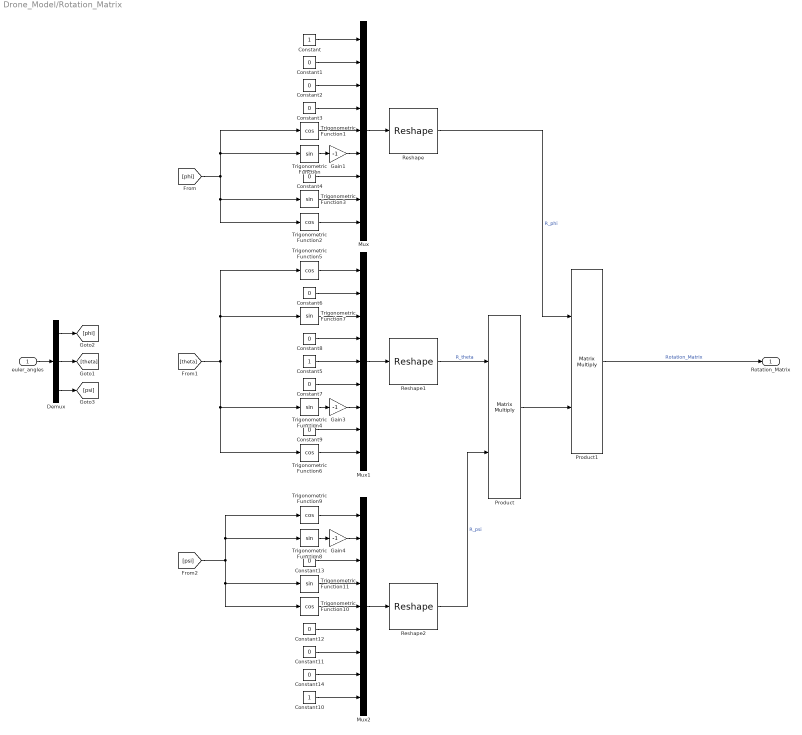
== system Drone_Model/Rotation_Matrix ==
  "euler_angles " : Inport
  Constant : Constant
  Constant{1..4,6..9,11..14} (12 alike) : Constant  Value=0
  Constant10 : Constant
  Constant5 : Constant
  Demux : Demux  Outputs=3
  Gain1 : Gain  Gain=-1
  Gain3 : Gain  Gain=-1
  Gain4 : Gain  Gain=-1
  Mux : Mux  Inputs=9
  Mux1 : Mux  Inputs=9
  Mux2 : Mux  Inputs=9
  Product : Product  Multiplication=Matrix(*)
  Product1 : Product  Multiplication=Matrix(*)
  Reshape : Reshape  OutputDimensionality=Customize  OutputDimensions=[3,3]
  Reshape1 : Reshape  OutputDimensionality=Customize  OutputDimensions=[3,3]
  Reshape2 : Reshape  OutputDimensionality=Customize  OutputDimensions=[3,3]
  Trigonometric Function{,3..4,7..8,11} (6 alike) : Trigonometry
  Trigonometric Function{1..2,5..6,9..10} (6 alike) : Trigonometry  Operator=cos
  Rotation_Matrix : Outport
  wires:
  Constant9/1 -> Mux1/8
  Constant11/1 -> Mux2/7
  Trigonometric Function1/1 -> Mux/5
  Trigonometric Function3/1 -> Mux/8
  Constant5/1 -> Mux1/5
  Trigonometric Function7/1 -> Mux1/3
  Reshape/1 -> Product1/1  "R_phi"
  Mux1/1 -> Reshape1/1
  Trigonometric Function8/1 -> Gain4/1
  Constant7/1 -> Mux1/6
  Trigonometric Function2/1 -> Mux/9
  [phi] -> Trigonometric Function2/1, Trigonometric Function3/1, Trigonometric Function1/1, Trigonometric Function/1
  Trigonometric Function6/1 -> Mux1/9
  Constant12/1 -> Mux2/6
  Trigonometric Function4/1 -> Gain3/1
  [theta] -> Trigonometric Function7/1, Trigonometric Function5/1, Trigonometric Function4/1, Trigonometric Function6/1
  Reshape2/1 -> Product/2  "R_psi"
  Trigonometric Function/1 -> Gain1/1
  Product/1 -> Product1/2
  Trigonometric Function5/1 -> Mux1/1
  Trigonometric Function9/1 -> Mux2/1
  Mux/1 -> Reshape/1
  Constant/1 -> Mux/1
  Constant3/1 -> Mux/4
  Constant6/1 -> Mux1/2
  Mux2/1 -> Reshape2/1
  Constant2/1 -> Mux/3
  Constant1/1 -> Mux/2
  [psi] -> Trigonometric Function11/1, Trigonometric Function10/1, Trigonometric Function9/1, Trigonometric Function8/1
  Constant8/1 -> Mux1/4
  Constant4/1 -> Mux/7
  Constant13/1 -> Mux2/3
  Trigonometric Function11/1 -> Mux2/4
  Constant10/1 -> Mux2/9
  Reshape1/1 -> Product/1  "R_theta"
  Constant14/1 -> Mux2/8
  Trigonometric Function10/1 -> Mux2/5
  Product1/1 -> Rotation_Matrix/1  "Rotation_Matrix"
  Demux/3 -> [psi]
  Demux/2 -> [theta]
  "euler_angles "/1 -> Demux/1
  Demux/1 -> [phi]
  Gain3/1 -> Mux1/7
  Gain1/1 -> Mux/6
  Gain4/1 -> Mux2/2

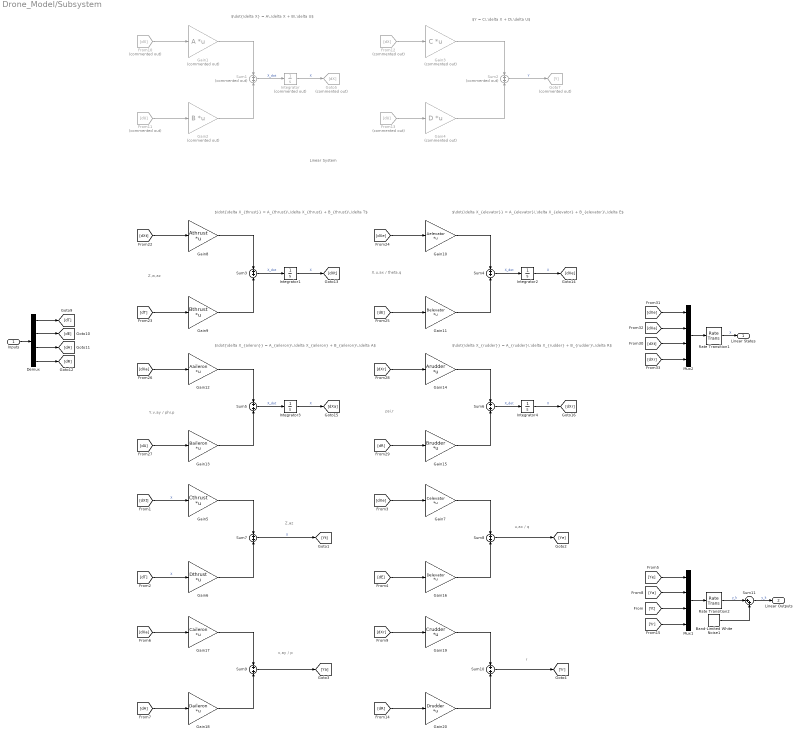
== system Drone_Model/Subsystem ==
  note: psi,r
  note: Y,v,ay / phi,p
  note: X,u,ax / theta,q
  note: Z,w,az
  note: Linear System
  note: $\dot{\delta X} = A\,\delta X + B\,\delta U$
  note: $Y = C\,\delta X + D\,\delta U$
  note: $\dot{\delta X_{thrust}} = A_{thrust}\,\delta X_{thrust} + B_{thrust}\,\delta T$
  note: $\dot{\delta X_{elevator}} = A_{elevator}\,\delta X_{elevator} + B_{elevator}\,\delta E$
  note: $\dot{\delta X_{aileron}} = A_{aileron}\,\delta X_{aileron} + B_{aileron}\,\delta A$
  note: $\dot{\delta X_{rudder}} = A_{rudder}\,\delta X_{rudder} + B_{rudder}\,\delta R$
  note: Z,az
  note: u,ax / q
  note: v,ay / p
  note: r
  "Inputs " : Inport
  Band-Limited White Noise1 : simulink/Sources/Band-Limited White Noise  Cov=[0.1;0.1;0.1;0.1;0.1;0.1;0.1;0.1;0.1]  Ts=0.05  seed=[11;12;13;14;15;16;17;18;19]
  Demux : Demux
  From10 : From  Commented=on  GotoTag=dX
  From11 : From  Commented=on  GotoTag=dU
  From12 : From  Commented=on  GotoTag=dX
  From13 : From  Commented=on  GotoTag=dU
  Gain1 : Gain  Commented=on  Gain=A  Multiplication=Matrix(K*u)
  Gain10 : Gain  Gain=Aelevator  Multiplication=Matrix(K*u)
  Gain11 : Gain  Gain=Belevator  Multiplication=Matrix(K*u)
  Gain12 : Gain  Gain=Aaileron  Multiplication=Matrix(K*u)
  Gain13 : Gain  Gain=Baileron  Multiplication=Matrix(K*u)
  Gain14 : Gain  Gain=Arudder  Multiplication=Matrix(K*u)
  Gain15 : Gain  Gain=Brudder  Multiplication=Matrix(K*u)
  Gain16 : Gain  Gain=Delevator  Multiplication=Matrix(K*u)
  Gain17 : Gain  Gain=Caileron  Multiplication=Matrix(K*u)
  Gain18 : Gain  Gain=Daileron  Multiplication=Matrix(K*u)
  Gain19 : Gain  Gain=Crudder  Multiplication=Matrix(K*u)
  Gain2 : Gain  Commented=on  Gain=B  Multiplication=Matrix(K*u)
  Gain20 : Gain  Gain=Drudder  Multiplication=Matrix(K*u)
  Gain3 : Gain  Commented=on  Gain=C  Multiplication=Matrix(K*u)
  Gain4 : Gain  Commented=on  Gain=D  Multiplication=Matrix(K*u)
  Gain5 : Gain  Gain=Cthrust  Multiplication=Matrix(K*u)
  Gain6 : Gain  Gain=Dthrust  Multiplication=Matrix(K*u)
  Gain7 : Gain  Gain=Celevator  Multiplication=Matrix(K*u)
  Gain8 : Gain  Gain=Athrust  Multiplication=Matrix(K*u)
  Gain9 : Gain  Gain=Bthrust  Multiplication=Matrix(K*u)
  Goto5 : Goto  Commented=on  GotoTag=dX
  Goto7 : Goto  Commented=on  GotoTag=Y
  Integrator : Integrator  Commented=on  InitialCondition=trim_state
  Integrator1 : Integrator  InitialCondition=trim_state(9:10)
  Integrator2 : Integrator  InitialCondition=trim_state(1:4)
  Integrator3 : Integrator  InitialCondition=trim_state(5:8)
  Integrator4 : Integrator  InitialCondition=trim_state(11:12)
  Mux1 : Mux
  Mux2 : Mux
  Rate Transition1 : RateTransition  OutPortSampleTime=0.005
  Rate Transition2 : RateTransition  OutPortSampleTime=0.005
  Sum1 : Sum  Commented=on  Inputs=+|+
  Sum{3..10} (8 alike) : Sum  Inputs=+|+
  Sum11 : Sum  Inputs=|++
  Sum2 : Sum  Commented=on  Inputs=+|+
  Linear States : Outport
  Linear Outputs : Outport  Port=2
  wires:
  Gain14/1 -> Sum6/1
  From11/1 -> Gain2/1
  [dXe] -> Gain10/1
  Gain10/1 -> Sum4/1
  Gain2/1 -> Sum1/2
  Gain15/1 -> Sum6/2
  Gain1/1 -> Sum1/1
  Sum5/1 -> Integrator3/1  "X_dot"
  Gain3/1 -> Sum2/1
  Integrator1/1 -> [dXt]  "X"
  From10/1 -> Gain1/1
  Sum1/1 -> Integrator/1  "X_dot"
  Sum2/1 -> Goto7/1  "Y"
  Integrator3/1 -> [dXa]  "X"
  Gain8/1 -> Sum3/1
  [dXt] -> Gain8/1
  Sum3/1 -> Integrator1/1  "X_dot"
  Integrator4/1 -> [dXr]  "X"
  Sum4/1 -> Integrator2/1  "X_dot"
  Gain13/1 -> Sum5/2
  [dXa] -> Gain12/1
  [dXr] -> Gain14/1
  Sum6/1 -> Integrator4/1  "X_dot"
  From13/1 -> Gain4/1
  Gain11/1 -> Sum4/2
  Integrator/1 -> Goto5/1  "X"
  Gain4/1 -> Sum2/2
  Gain12/1 -> Sum5/1
  Integrator2/1 -> [dXe]  "X"
  From12/1 -> Gain3/1
  "Inputs "/1 -> Demux/1
  Demux/3 -> [dA]
  Demux/2 -> [dE]
  Demux/1 -> [dT]
  Demux/4 -> [dR]
  [dXt] -> Mux2/3
  [dXr] -> Mux2/4
  Mux2/1 -> Rate Transition1/1
  [dXe] -> Mux2/1
  [dXa] -> Mux2/2
  Gain6/1 -> Sum7/2
  Gain5/1 -> Sum7/1
  Gain16/1 -> Sum8/2
  [dE] -> Gain16/1
  Gain7/1 -> Sum8/1
  [dXe] -> Gain7/1
  [dA] -> Gain18/1
  Gain17/1 -> Sum9/1
  [dXa] -> Gain17/1
  Gain18/1 -> Sum9/2
  [dXr] -> Gain19/1
  [dR] -> Gain20/1
  Gain20/1 -> Sum10/2
  Gain19/1 -> Sum10/1
  [Ya] -> Mux1/2
  [Ye] -> Mux1/1
  Mux1/1 -> Rate Transition2/1
  [Yr] -> Mux1/4
  [Yt] -> Mux1/3
  [dT] -> Gain9/1
  [dA] -> Gain13/1
  [dR] -> Gain15/1
  [dE] -> Gain11/1
  Sum9/1 -> [Ya]
  Sum10/1 -> [Yr]
  Sum8/1 -> [Ye]
  Sum11/1 -> Linear Outputs/1  "y_k"
  Gain9/1 -> Sum3/2
  [dT] -> Gain6/1  "X"
  [dXt] -> Gain5/1  "X"
  Sum7/1 -> [Yt]  "X"
  Rate Transition1/1 -> Linear States/1  "X"
  Band-Limited White Noise1/1 -> Sum11/2
  Rate Transition2/1 -> Sum11/1  "y_k"

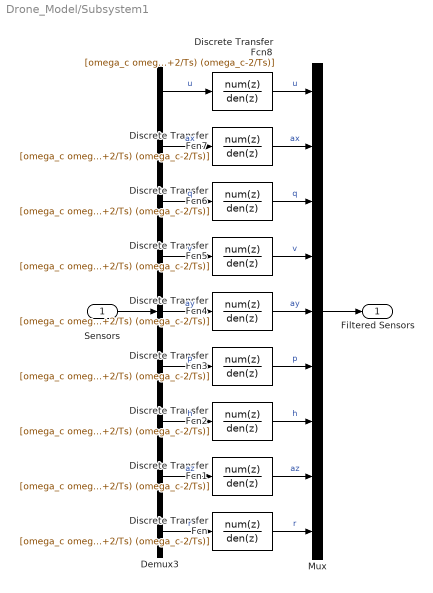
== system Drone_Model/Subsystem1 ==
  Sensors : Inport
  Demux3 : Demux  Outputs=9
  Discrete Transfer Fcn{,1..8} (9 alike) : DiscreteTransferFcn  Numerator=[omega_c omega_c]  Denominator=[(omega_c+2/Ts) (omega_c-2/Ts)]  SampleTime=0.005
  Mux : Mux  Inputs=9
  Filtered Sensors : Outport
  wires:
  Demux3/6 -> Discrete Transfer Fcn3/1  "p"
  Demux3/5 -> Discrete Transfer Fcn4/1  "ay"
  Demux3/7 -> Discrete Transfer Fcn2/1  "h"
  Demux3/4 -> Discrete Transfer Fcn5/1  "v"
  Demux3/9 -> Discrete Transfer Fcn/1  "r"
  Demux3/8 -> Discrete Transfer Fcn1/1  "az"
  Demux3/2 -> Discrete Transfer Fcn7/1  "ax"
  Sensors/1 -> Demux3/1
  Demux3/3 -> Discrete Transfer Fcn6/1  "q"
  Demux3/1 -> Discrete Transfer Fcn8/1  "u"
  Discrete Transfer Fcn/1 -> Mux/9  "r"
  Discrete Transfer Fcn1/1 -> Mux/8  "az"
  Discrete Transfer Fcn2/1 -> Mux/7  "h"
  Discrete Transfer Fcn3/1 -> Mux/6  "p"
  Discrete Transfer Fcn4/1 -> Mux/5  "ay"
  Discrete Transfer Fcn5/1 -> Mux/4  "v"
  Discrete Transfer Fcn6/1 -> Mux/3  "q"
  Discrete Transfer Fcn7/1 -> Mux/2  "ax"
  Discrete Transfer Fcn8/1 -> Mux/1  "u"
  Mux/1 -> Filtered Sensors/1

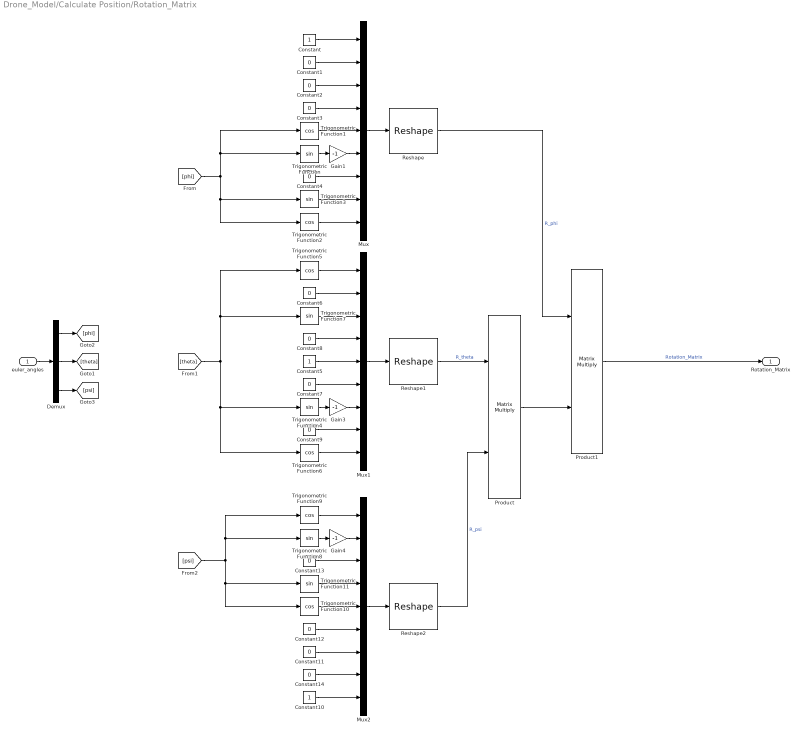
== system Drone_Model/Calculate Position/Rotation_Matrix ==
  "euler_angles " : Inport
  Constant : Constant
  Constant{1..4,6..9,11..14} (12 alike) : Constant  Value=0
  Constant10 : Constant
  Constant5 : Constant
  Demux : Demux  Outputs=3
  Gain1 : Gain  Gain=-1
  Gain3 : Gain  Gain=-1
  Gain4 : Gain  Gain=-1
  Mux : Mux  Inputs=9
  Mux1 : Mux  Inputs=9
  Mux2 : Mux  Inputs=9
  Product : Product  Multiplication=Matrix(*)
  Product1 : Product  Multiplication=Matrix(*)
  Reshape : Reshape  OutputDimensionality=Customize  OutputDimensions=[3,3]
  Reshape1 : Reshape  OutputDimensionality=Customize  OutputDimensions=[3,3]
  Reshape2 : Reshape  OutputDimensionality=Customize  OutputDimensions=[3,3]
  Trigonometric Function{,3..4,7..8,11} (6 alike) : Trigonometry
  Trigonometric Function{1..2,5..6,9..10} (6 alike) : Trigonometry  Operator=cos
  Rotation_Matrix : Outport
  wires:
  Constant9/1 -> Mux1/8
  Constant11/1 -> Mux2/7
  Trigonometric Function1/1 -> Mux/5
  Trigonometric Function3/1 -> Mux/8
  Constant5/1 -> Mux1/5
  Trigonometric Function7/1 -> Mux1/3
  Reshape/1 -> Product1/1  "R_phi"
  Mux1/1 -> Reshape1/1
  Trigonometric Function8/1 -> Gain4/1
  Constant7/1 -> Mux1/6
  Trigonometric Function2/1 -> Mux/9
  [phi] -> Trigonometric Function2/1, Trigonometric Function3/1, Trigonometric Function1/1, Trigonometric Function/1
  Trigonometric Function6/1 -> Mux1/9
  Constant12/1 -> Mux2/6
  Trigonometric Function4/1 -> Gain3/1
  [theta] -> Trigonometric Function7/1, Trigonometric Function5/1, Trigonometric Function4/1, Trigonometric Function6/1
  Reshape2/1 -> Product/2  "R_psi"
  Trigonometric Function/1 -> Gain1/1
  Product/1 -> Product1/2
  Trigonometric Function5/1 -> Mux1/1
  Trigonometric Function9/1 -> Mux2/1
  Mux/1 -> Reshape/1
  Constant/1 -> Mux/1
  Constant3/1 -> Mux/4
  Constant6/1 -> Mux1/2
  Mux2/1 -> Reshape2/1
  Constant2/1 -> Mux/3
  Constant1/1 -> Mux/2
  [psi] -> Trigonometric Function11/1, Trigonometric Function10/1, Trigonometric Function9/1, Trigonometric Function8/1
  Constant8/1 -> Mux1/4
  Constant4/1 -> Mux/7
  Constant13/1 -> Mux2/3
  Trigonometric Function11/1 -> Mux2/4
  Constant10/1 -> Mux2/9
  Reshape1/1 -> Product/1  "R_theta"
  Constant14/1 -> Mux2/8
  Trigonometric Function10/1 -> Mux2/5
  Product1/1 -> Rotation_Matrix/1  "Rotation_Matrix"
  Demux/3 -> [psi]
  Demux/2 -> [theta]
  "euler_angles "/1 -> Demux/1
  Demux/1 -> [phi]
  Gain3/1 -> Mux1/7
  Gain1/1 -> Mux/6
  Gain4/1 -> Mux2/2

== system Drone_Model/Calculate Velocity/Calculate_Thrust ==
  note: $F_{T} = \sum_{i=1}^4[0;0;C_{T}.*n.^2]$
  n : Inport
  Constant15 : Constant  Value=C_T(1)
  Constant16 : Constant  Value=2
  Gain4 : Gain  Gain=Thrust_Sum  Multiplication=Matrix(K*u)
      settings: AttributesFormatString=%<Gain>
  Gain5 : Gain  Gain=C_T(2)
  Power : Math  Operator=pow  SignedPower=off  SaturateOnIntegerOverflow=on
  Product2 : Product
  Sum1 : Sum  Inputs=++|
  F_T : Outport
  wires:
  Constant15/1 -> Sum1/1
  Gain4/1 -> F_T/1  "F_T"
  n/1 -> Power/1, Gain5/1
  Power/1 -> Product2/2  "props squared"
  Gain5/1 -> Sum1/2
  Sum1/1 -> Product2/1
  Product2/1 -> Gain4/1
  Constant16/1 -> Power/2

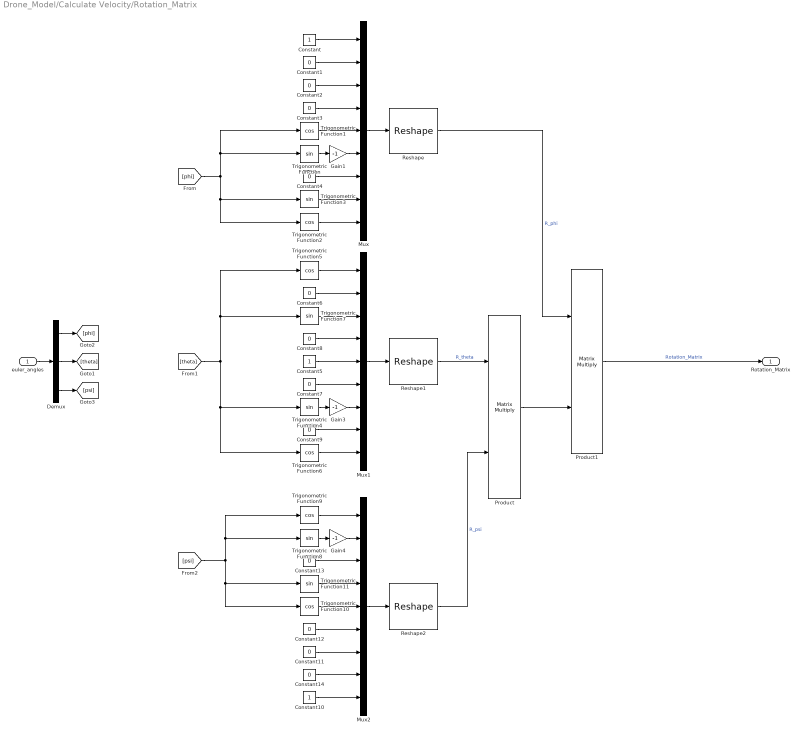
== system Drone_Model/Calculate Velocity/Rotation_Matrix ==
  "euler_angles " : Inport
  Constant : Constant
  Constant{1..4,6..9,11..14} (12 alike) : Constant  Value=0
  Constant10 : Constant
  Constant5 : Constant
  Demux : Demux  Outputs=3
  Gain1 : Gain  Gain=-1
  Gain3 : Gain  Gain=-1
  Gain4 : Gain  Gain=-1
  Mux : Mux  Inputs=9
  Mux1 : Mux  Inputs=9
  Mux2 : Mux  Inputs=9
  Product : Product  Multiplication=Matrix(*)
  Product1 : Product  Multiplication=Matrix(*)
  Reshape : Reshape  OutputDimensionality=Customize  OutputDimensions=[3,3]
  Reshape1 : Reshape  OutputDimensionality=Customize  OutputDimensions=[3,3]
  Reshape2 : Reshape  OutputDimensionality=Customize  OutputDimensions=[3,3]
  Trigonometric Function{,3..4,7..8,11} (6 alike) : Trigonometry
  Trigonometric Function{1..2,5..6,9..10} (6 alike) : Trigonometry  Operator=cos
  Rotation_Matrix : Outport
  wires:
  Constant9/1 -> Mux1/8
  Constant11/1 -> Mux2/7
  Trigonometric Function1/1 -> Mux/5
  Trigonometric Function3/1 -> Mux/8
  Constant5/1 -> Mux1/5
  Trigonometric Function7/1 -> Mux1/3
  Reshape/1 -> Product1/1  "R_phi"
  Mux1/1 -> Reshape1/1
  Trigonometric Function8/1 -> Gain4/1
  Constant7/1 -> Mux1/6
  Trigonometric Function2/1 -> Mux/9
  [phi] -> Trigonometric Function2/1, Trigonometric Function3/1, Trigonometric Function1/1, Trigonometric Function/1
  Trigonometric Function6/1 -> Mux1/9
  Constant12/1 -> Mux2/6
  Trigonometric Function4/1 -> Gain3/1
  [theta] -> Trigonometric Function7/1, Trigonometric Function5/1, Trigonometric Function4/1, Trigonometric Function6/1
  Reshape2/1 -> Product/2  "R_psi"
  Trigonometric Function/1 -> Gain1/1
  Product/1 -> Product1/2
  Trigonometric Function5/1 -> Mux1/1
  Trigonometric Function9/1 -> Mux2/1
  Mux/1 -> Reshape/1
  Constant/1 -> Mux/1
  Constant3/1 -> Mux/4
  Constant6/1 -> Mux1/2
  Mux2/1 -> Reshape2/1
  Constant2/1 -> Mux/3
  Constant1/1 -> Mux/2
  [psi] -> Trigonometric Function11/1, Trigonometric Function10/1, Trigonometric Function9/1, Trigonometric Function8/1
  Constant8/1 -> Mux1/4
  Constant4/1 -> Mux/7
  Constant13/1 -> Mux2/3
  Trigonometric Function11/1 -> Mux2/4
  Constant10/1 -> Mux2/9
  Reshape1/1 -> Product/1  "R_theta"
  Constant14/1 -> Mux2/8
  Trigonometric Function10/1 -> Mux2/5
  Product1/1 -> Rotation_Matrix/1  "Rotation_Matrix"
  Demux/3 -> [psi]
  Demux/2 -> [theta]
  "euler_angles "/1 -> Demux/1
  Demux/1 -> [phi]
  Gain3/1 -> Mux1/7
  Gain1/1 -> Mux/6
  Gain4/1 -> Mux2/2
